simulink model "Carrito_B"  (R2013a)
settings: Solver=ode113  StartTime=0.0  StopTime=10  RelTol=1e-3
InitFcn:
  | M=0.2;m=0.1;l=0.3;B1=0;B2=0;g=-9.81;
StartFcn:
  | M=0.2;m=0.1;l=0.3;B1=0;B2=0;g=-9.81;
settings Model: Creator=LuisFernando  LastModifiedBy=LuisFernando

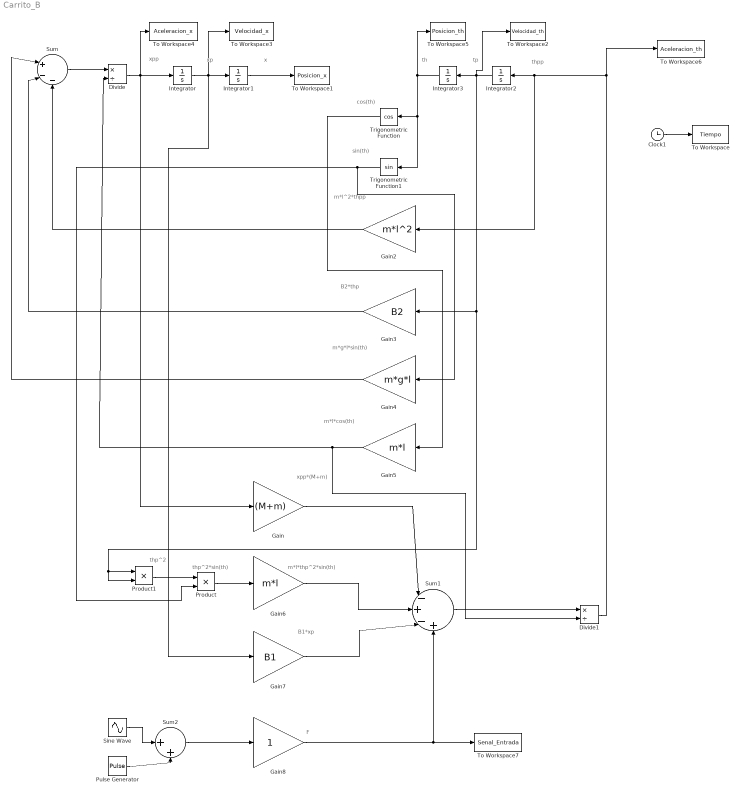
== system Carrito_B ==
  note: B1*xp
  note: F
  note: xpp*(M+m)
  note: m*l*thp^2*sin(th)
  note: thp^2*sin(th)
  note: thp^2
  note: m*l*cos(th)
  note: m*l^2*thpp
  note: sin(th)
  note: cos(th)
  note: xpp
  note: x
  note: xp
  note: thpp
  note: th
  note: tp
  note: B2*thp
  note: m*g*l*sin(th)
  Clock1 : Clock
      settings: Decimation=100
  Divide : Product  Inputs=*/
  Divide1 : Product  Inputs=*/
  Gain : Gain  Gain=(M+m)
  Gain2 : Gain  Gain=m*l^2
  Gain3 : Gain  Gain=B2
  Gain4 : Gain  Gain=m*g*l
  Gain5 : Gain  Gain=m*l
  Gain6 : Gain  Gain=m*l
  Gain7 : Gain  Gain=B1
  Gain8 : Gain
  Integrator{,1..3} (4 alike) : Integrator
  Product : Product
  Product1 : Product
  Pulse Generator : DiscretePulseGenerator  PulseType=Time based  Amplitude=15  PulseWidth=50
  Sine Wave : Sin  Amplitude=0  SampleTime=0
  Sum : Sum  Inputs=|+--
  Sum1 : Sum  Inputs=|-+-+
  Sum2 : Sum  Inputs=|++
  To Workspace : ToWorkspace  VariableName=Tiempo  SampleTime=0.01
  To Workspace1 : ToWorkspace  VariableName=Posicion_x  SampleTime=0.01
  To Workspace2 : ToWorkspace  VariableName=Velocidad_th  SampleTime=0.01
  To Workspace3 : ToWorkspace  VariableName=Velocidad_x  SampleTime=0.01
  To Workspace4 : ToWorkspace  VariableName=Aceleracion_x  SampleTime=0.01
  To Workspace5 : ToWorkspace  VariableName=Posicion_th  SampleTime=0.01
  To Workspace6 : ToWorkspace  VariableName=Aceleracion_th  SampleTime=0.01
  To Workspace7 : ToWorkspace  VariableName=Senal_Entrada  SampleTime=0.01
  Trigonometric Function : Trigonometry  Operator=cos
  Trigonometric Function1 : Trigonometry
  wires:
  Integrator/1 -> Integrator1/1, To Workspace3/1, Gain7/1
  Divide1/1 -> To Workspace6/1, Gain2/1, Integrator2/1
  Integrator3/1 -> Trigonometric Function1/1, Trigonometric Function/1, To Workspace5/1
  Trigonometric Function1/1 -> Product/2, Gain4/1
  Trigonometric Function/1 -> Gain5/1
  Sum/1 -> Divide/1
  Gain2/1 -> Sum/3
  Gain3/1 -> Sum/2
  Gain4/1 -> Sum/1
  Divide/1 -> To Workspace4/1, Gain/1, Integrator/1
  Product1/1 -> Product/1
  Integrator2/1 -> Product1/2, Product1/1, Gain3/1, To Workspace2/1, Integrator3/1
  Product/1 -> Gain6/1
  Gain/1 -> Sum1/1
  Gain6/1 -> Sum1/2
  Gain7/1 -> Sum1/3
  Sine Wave/1 -> Sum2/1
  Pulse Generator/1 -> Sum2/2
  Sum2/1 -> Gain8/1
  Gain8/1 -> To Workspace7/1, Sum1/4
  Sum1/1 -> Divide1/1
  Gain5/1 -> Divide/2, Divide1/2
  Clock1/1 -> To Workspace/1
  Integrator1/1 -> To Workspace1/1
